simulink model "tesv"  (R2012b)
settings: Solver=ode45  SolverMode=SingleTasking  StartTime=0.0  StopTime=10.0  RelTol=1e-3
libraries: xbsIndex_r4 x837
(part 2 of 6)

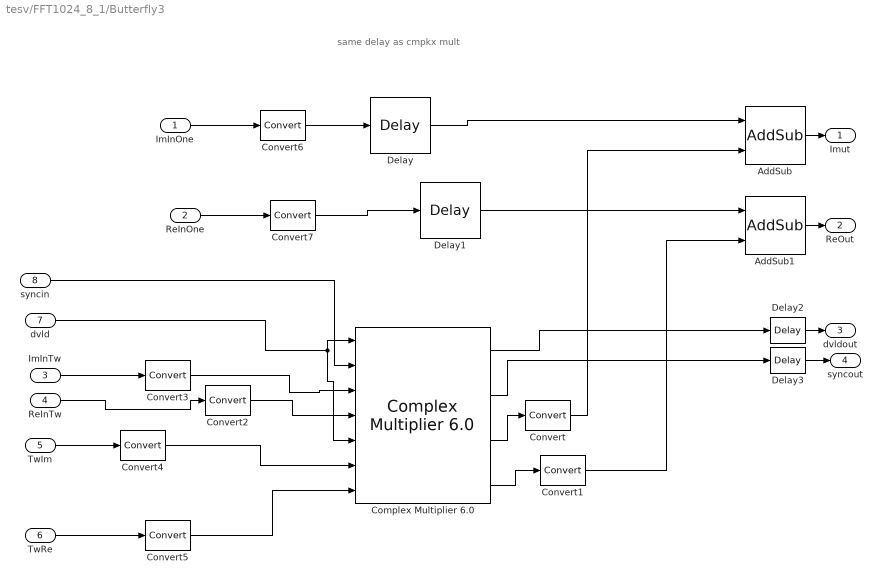
== system tesv/FFT1024_8_1/Butterfly3 ==
  note: same delay as cmpkx mult
  ImInOne : Inport
  ReInOne : Inport  Port=2
  ImInTw : Inport  Port=3
  ReInTw : Inport  Port=4
  TwIm : Inport  Port=5
  TwRe : Inport  Port=6
  dvld : Inport  Port=7
  syncin : Inport  Port=8
  AddSub : xbsIndex_r4/AddSub  mode=Addition  use_carryin=off  use_carryout=off  en=off  latency=1  precision=Full  arith_type=Unsigned  n_bits=16  bin_pt=14  quantization=Truncate  overflow=Wrap  use_behavioral_HDL=off  hw_selection=Fabric  pipelined=off  dbl_ovrd=off  block_type=addsub
  AddSub1 : xbsIndex_r4/AddSub  mode=Addition  use_carryin=off  use_carryout=off  en=off  latency=1  precision=Full  arith_type=Unsigned  n_bits=16  bin_pt=14  quantization=Truncate  overflow=Wrap  use_behavioral_HDL=off  hw_selection=Fabric  pipelined=off  dbl_ovrd=off  block_type=addsub
  "Complex Multiplier 6.0 " : xbsIndex_r4/Complex Multiplier 6.0   hasatlast=on  hasatuser=off  atuserwidth=1  hasbtlast=off  hasbtuser=off  btuserwidth=1  multtype=Use_Mults  optimizegoal=Resources  flowcontrol=NonBlocking  outputwidth=18  roundmode=Truncate  hasctrltlast=off  hasctrltuser=off  ctrltuserwidth=1  outtlastbehv=Pass_A_TLAST  latencyconfig=Automatic  minimumlatency=37  aclken=off  aresetn=off  trim_axipin_name=on  simulation_type=hybrid_sim  simulation_model=sysgen:cmpy_v6_0  data_path_portlist={ 's_axis_a_tdata_real', 's_axis_a_tdata_imag', 's_axis_b_tdata_real', 's_axis_b_tdata_imag', 's_axis_ctrl_tdata_rounding_bit', 'm_axis_dout_tdata_real', 'm_axis_dout_tdata_imag' }  aportwidth=63  bportwidth=63  ip_name=Complex Multiplier  ip_version=6.0  dsptool_ready=true  ipcore_usecache=true  ipcore_useipmodelcache=true  ipcore_verbose=false  ipcore_latency_parameter='minimumlatency'  wrapper_available=true  port_translation_map={ 'aclken' => 'en', 'aresetn' => 'rst'}  block_type=cmpy_v6_0
  Convert{,1..7} (8 alike) : xbsIndex_r4/Convert  gui_display_data_type=Fixed-point  arith_type="Signed  (2's comp)"  n_bits=16  bin_pt=14  float_type=Single  exp_bits=8  fraction_bits=24  quantization=Truncate  overflow=Wrap  en=off  latency=0  pipeline=off  dbl_ovrd=off  block_type=convert
  Delay : xbsIndex_r4/Delay  rst=off  infoeditControl=Selection of Reset will increase slice count due to use of real FFs and instead of SRLs  en=off  latency=6  reg_retiming=off  dbl_ovrd=off  block_type=delay
  Delay1 : xbsIndex_r4/Delay  rst=off  infoeditControl=Selection of Reset will increase slice count due to use of real FFs and instead of SRLs  en=off  latency=6  reg_retiming=off  dbl_ovrd=off  block_type=delay
  Delay2 : xbsIndex_r4/Delay  rst=off  infoeditControl=Selection of Reset will increase slice count due to use of real FFs and instead of SRLs  en=off  latency=1  reg_retiming=off  dbl_ovrd=off  block_type=delay
  Delay3 : xbsIndex_r4/Delay  rst=off  infoeditControl=Selection of Reset will increase slice count due to use of real FFs and instead of SRLs  en=off  latency=1  reg_retiming=off  dbl_ovrd=off  block_type=delay
  Imut : Outport
  ReOut : Outport  Port=2
  dvldout : Outport  Port=3
  syncout : Outport  Port=4
  wires:
  ReInOne/1 -> Convert7/1
  ImInOne/1 -> Convert6/1
  AddSub/1 -> Imut/1
  AddSub1/1 -> ReOut/1
  ImInTw/1 -> Convert3/1
  ReInTw/1 -> Convert2/1
  Delay/1 -> AddSub/1
  Delay1/1 -> AddSub1/1
  TwIm/1 -> Convert4/1
  TwRe/1 -> Convert5/1
  dvld/1 -> "Complex Multiplier 6.0 "/1, "Complex Multiplier 6.0 "/5
  Convert6/1 -> Delay/1
  Convert7/1 -> Delay1/1
  Convert3/1 -> "Complex Multiplier 6.0 "/3
  Convert2/1 -> "Complex Multiplier 6.0 "/4
  Convert4/1 -> "Complex Multiplier 6.0 "/6
  Convert5/1 -> "Complex Multiplier 6.0 "/7
  Convert1/1 -> AddSub1/2
  syncin/1 -> "Complex Multiplier 6.0 "/2
  "Complex Multiplier 6.0 "/4 -> Convert1/1
  "Complex Multiplier 6.0 "/3 -> Convert/1
  "Complex Multiplier 6.0 "/1 -> Delay2/1
  "Complex Multiplier 6.0 "/2 -> Delay3/1
  Convert/1 -> AddSub/2
  Delay2/1 -> dvldout/1
  Delay3/1 -> syncout/1

== system tesv/FFT1024_8_1/Butterfly4 ==
  note: same delay as cmpkx mult
  ImInOne : Inport
  ReInOne : Inport  Port=2
  ImInTw : Inport  Port=3
  ReInTw : Inport  Port=4
  TwIm : Inport  Port=5
  TwRe : Inport  Port=6
  dvld : Inport  Port=7
  syncin : Inport  Port=8
  AddSub : xbsIndex_r4/AddSub  mode=Addition  use_carryin=off  use_carryout=off  en=off  latency=1  precision=Full  arith_type=Unsigned  n_bits=16  bin_pt=14  quantization=Truncate  overflow=Wrap  use_behavioral_HDL=off  hw_selection=Fabric  pipelined=off  dbl_ovrd=off  block_type=addsub
  AddSub1 : xbsIndex_r4/AddSub  mode=Addition  use_carryin=off  use_carryout=off  en=off  latency=1  precision=Full  arith_type=Unsigned  n_bits=16  bin_pt=14  quantization=Truncate  overflow=Wrap  use_behavioral_HDL=off  hw_selection=Fabric  pipelined=off  dbl_ovrd=off  block_type=addsub
  "Complex Multiplier 6.0 " : xbsIndex_r4/Complex Multiplier 6.0   hasatlast=on  hasatuser=off  atuserwidth=1  hasbtlast=off  hasbtuser=off  btuserwidth=1  multtype=Use_Mults  optimizegoal=Resources  flowcontrol=NonBlocking  outputwidth=18  roundmode=Truncate  hasctrltlast=off  hasctrltuser=off  ctrltuserwidth=1  outtlastbehv=Pass_A_TLAST  latencyconfig=Automatic  minimumlatency=37  aclken=off  aresetn=off  trim_axipin_name=on  simulation_type=hybrid_sim  simulation_model=sysgen:cmpy_v6_0  data_path_portlist={ 's_axis_a_tdata_real', 's_axis_a_tdata_imag', 's_axis_b_tdata_real', 's_axis_b_tdata_imag', 's_axis_ctrl_tdata_rounding_bit', 'm_axis_dout_tdata_real', 'm_axis_dout_tdata_imag' }  aportwidth=63  bportwidth=63  ip_name=Complex Multiplier  ip_version=6.0  dsptool_ready=true  ipcore_usecache=true  ipcore_useipmodelcache=true  ipcore_verbose=false  ipcore_latency_parameter='minimumlatency'  wrapper_available=true  port_translation_map={ 'aclken' => 'en', 'aresetn' => 'rst'}  block_type=cmpy_v6_0
  Convert{,1..7} (8 alike) : xbsIndex_r4/Convert  gui_display_data_type=Fixed-point  arith_type="Signed  (2's comp)"  n_bits=16  bin_pt=14  float_type=Single  exp_bits=8  fraction_bits=24  quantization=Truncate  overflow=Wrap  en=off  latency=0  pipeline=off  dbl_ovrd=off  block_type=convert
  Delay : xbsIndex_r4/Delay  rst=off  infoeditControl=Selection of Reset will increase slice count due to use of real FFs and instead of SRLs  en=off  latency=6  reg_retiming=off  dbl_ovrd=off  block_type=delay
  Delay1 : xbsIndex_r4/Delay  rst=off  infoeditControl=Selection of Reset will increase slice count due to use of real FFs and instead of SRLs  en=off  latency=6  reg_retiming=off  dbl_ovrd=off  block_type=delay
  Delay2 : xbsIndex_r4/Delay  rst=off  infoeditControl=Selection of Reset will increase slice count due to use of real FFs and instead of SRLs  en=off  latency=1  reg_retiming=off  dbl_ovrd=off  block_type=delay
  Delay3 : xbsIndex_r4/Delay  rst=off  infoeditControl=Selection of Reset will increase slice count due to use of real FFs and instead of SRLs  en=off  latency=1  reg_retiming=off  dbl_ovrd=off  block_type=delay
  Imut : Outport
  ReOut : Outport  Port=2
  dvldout : Outport  Port=3
  syncout : Outport  Port=4
  wires:
  ReInOne/1 -> Convert7/1
  ImInOne/1 -> Convert6/1
  AddSub/1 -> Imut/1
  AddSub1/1 -> ReOut/1
  ImInTw/1 -> Convert3/1
  ReInTw/1 -> Convert2/1
  Delay/1 -> AddSub/1
  Delay1/1 -> AddSub1/1
  TwIm/1 -> Convert4/1
  TwRe/1 -> Convert5/1
  dvld/1 -> "Complex Multiplier 6.0 "/1, "Complex Multiplier 6.0 "/5
  Convert6/1 -> Delay/1
  Convert7/1 -> Delay1/1
  Convert3/1 -> "Complex Multiplier 6.0 "/3
  Convert2/1 -> "Complex Multiplier 6.0 "/4
  Convert4/1 -> "Complex Multiplier 6.0 "/6
  Convert5/1 -> "Complex Multiplier 6.0 "/7
  Convert1/1 -> AddSub1/2
  syncin/1 -> "Complex Multiplier 6.0 "/2
  "Complex Multiplier 6.0 "/4 -> Convert1/1
  "Complex Multiplier 6.0 "/3 -> Convert/1
  "Complex Multiplier 6.0 "/1 -> Delay2/1
  "Complex Multiplier 6.0 "/2 -> Delay3/1
  Convert/1 -> AddSub/2
  Delay2/1 -> dvldout/1
  Delay3/1 -> syncout/1

== system tesv/FFT1024_8_1/Butterfly5 ==
  note: same delay as cmpkx mult
  ImInOne : Inport
  ReInOne : Inport  Port=2
  ImInTw : Inport  Port=3
  ReInTw : Inport  Port=4
  TwIm : Inport  Port=5
  TwRe : Inport  Port=6
  dvld : Inport  Port=7
  syncin : Inport  Port=8
  AddSub : xbsIndex_r4/AddSub  mode=Addition  use_carryin=off  use_carryout=off  en=off  latency=1  precision=Full  arith_type=Unsigned  n_bits=16  bin_pt=14  quantization=Truncate  overflow=Wrap  use_behavioral_HDL=off  hw_selection=Fabric  pipelined=off  dbl_ovrd=off  block_type=addsub
  AddSub1 : xbsIndex_r4/AddSub  mode=Addition  use_carryin=off  use_carryout=off  en=off  latency=1  precision=Full  arith_type=Unsigned  n_bits=16  bin_pt=14  quantization=Truncate  overflow=Wrap  use_behavioral_HDL=off  hw_selection=Fabric  pipelined=off  dbl_ovrd=off  block_type=addsub
  "Complex Multiplier 6.0 " : xbsIndex_r4/Complex Multiplier 6.0   hasatlast=on  hasatuser=off  atuserwidth=1  hasbtlast=off  hasbtuser=off  btuserwidth=1  multtype=Use_Mults  optimizegoal=Resources  flowcontrol=NonBlocking  outputwidth=18  roundmode=Truncate  hasctrltlast=off  hasctrltuser=off  ctrltuserwidth=1  outtlastbehv=Pass_A_TLAST  latencyconfig=Automatic  minimumlatency=37  aclken=off  aresetn=off  trim_axipin_name=on  simulation_type=hybrid_sim  simulation_model=sysgen:cmpy_v6_0  data_path_portlist={ 's_axis_a_tdata_real', 's_axis_a_tdata_imag', 's_axis_b_tdata_real', 's_axis_b_tdata_imag', 's_axis_ctrl_tdata_rounding_bit', 'm_axis_dout_tdata_real', 'm_axis_dout_tdata_imag' }  aportwidth=63  bportwidth=63  ip_name=Complex Multiplier  ip_version=6.0  dsptool_ready=true  ipcore_usecache=true  ipcore_useipmodelcache=true  ipcore_verbose=false  ipcore_latency_parameter='minimumlatency'  wrapper_available=true  port_translation_map={ 'aclken' => 'en', 'aresetn' => 'rst'}  block_type=cmpy_v6_0
  Convert{,1..7} (8 alike) : xbsIndex_r4/Convert  gui_display_data_type=Fixed-point  arith_type="Signed  (2's comp)"  n_bits=16  bin_pt=14  float_type=Single  exp_bits=8  fraction_bits=24  quantization=Truncate  overflow=Wrap  en=off  latency=0  pipeline=off  dbl_ovrd=off  block_type=convert
  Delay : xbsIndex_r4/Delay  rst=off  infoeditControl=Selection of Reset will increase slice count due to use of real FFs and instead of SRLs  en=off  latency=6  reg_retiming=off  dbl_ovrd=off  block_type=delay
  Delay1 : xbsIndex_r4/Delay  rst=off  infoeditControl=Selection of Reset will increase slice count due to use of real FFs and instead of SRLs  en=off  latency=6  reg_retiming=off  dbl_ovrd=off  block_type=delay
  Delay2 : xbsIndex_r4/Delay  rst=off  infoeditControl=Selection of Reset will increase slice count due to use of real FFs and instead of SRLs  en=off  latency=1  reg_retiming=off  dbl_ovrd=off  block_type=delay
  Delay3 : xbsIndex_r4/Delay  rst=off  infoeditControl=Selection of Reset will increase slice count due to use of real FFs and instead of SRLs  en=off  latency=1  reg_retiming=off  dbl_ovrd=off  block_type=delay
  Imut : Outport
  ReOut : Outport  Port=2
  dvldout : Outport  Port=3
  syncout : Outport  Port=4
  wires:
  ReInOne/1 -> Convert7/1
  ImInOne/1 -> Convert6/1
  AddSub/1 -> Imut/1
  AddSub1/1 -> ReOut/1
  ImInTw/1 -> Convert3/1
  ReInTw/1 -> Convert2/1
  Delay/1 -> AddSub/1
  Delay1/1 -> AddSub1/1
  TwIm/1 -> Convert4/1
  TwRe/1 -> Convert5/1
  dvld/1 -> "Complex Multiplier 6.0 "/1, "Complex Multiplier 6.0 "/5
  Convert6/1 -> Delay/1
  Convert7/1 -> Delay1/1
  Convert3/1 -> "Complex Multiplier 6.0 "/3
  Convert2/1 -> "Complex Multiplier 6.0 "/4
  Convert4/1 -> "Complex Multiplier 6.0 "/6
  Convert5/1 -> "Complex Multiplier 6.0 "/7
  Convert1/1 -> AddSub1/2
  syncin/1 -> "Complex Multiplier 6.0 "/2
  "Complex Multiplier 6.0 "/4 -> Convert1/1
  "Complex Multiplier 6.0 "/3 -> Convert/1
  "Complex Multiplier 6.0 "/1 -> Delay2/1
  "Complex Multiplier 6.0 "/2 -> Delay3/1
  Convert/1 -> AddSub/2
  Delay2/1 -> dvldout/1
  Delay3/1 -> syncout/1

== system tesv/FFT1024_8_1/Butterfly6 ==
  note: same delay as cmpkx mult
  ImInOne : Inport
  ReInOne : Inport  Port=2
  ImInTw : Inport  Port=3
  ReInTw : Inport  Port=4
  TwIm : Inport  Port=5
  TwRe : Inport  Port=6
  dvld : Inport  Port=7
  syncin : Inport  Port=8
  AddSub : xbsIndex_r4/AddSub  mode=Addition  use_carryin=off  use_carryout=off  en=off  latency=1  precision=Full  arith_type=Unsigned  n_bits=16  bin_pt=14  quantization=Truncate  overflow=Wrap  use_behavioral_HDL=off  hw_selection=Fabric  pipelined=off  dbl_ovrd=off  block_type=addsub
  AddSub1 : xbsIndex_r4/AddSub  mode=Addition  use_carryin=off  use_carryout=off  en=off  latency=1  precision=Full  arith_type=Unsigned  n_bits=16  bin_pt=14  quantization=Truncate  overflow=Wrap  use_behavioral_HDL=off  hw_selection=Fabric  pipelined=off  dbl_ovrd=off  block_type=addsub
  "Complex Multiplier 6.0 " : xbsIndex_r4/Complex Multiplier 6.0   hasatlast=on  hasatuser=off  atuserwidth=1  hasbtlast=off  hasbtuser=off  btuserwidth=1  multtype=Use_Mults  optimizegoal=Resources  flowcontrol=NonBlocking  outputwidth=18  roundmode=Truncate  hasctrltlast=off  hasctrltuser=off  ctrltuserwidth=1  outtlastbehv=Pass_A_TLAST  latencyconfig=Automatic  minimumlatency=37  aclken=off  aresetn=off  trim_axipin_name=on  simulation_type=hybrid_sim  simulation_model=sysgen:cmpy_v6_0  data_path_portlist={ 's_axis_a_tdata_real', 's_axis_a_tdata_imag', 's_axis_b_tdata_real', 's_axis_b_tdata_imag', 's_axis_ctrl_tdata_rounding_bit', 'm_axis_dout_tdata_real', 'm_axis_dout_tdata_imag' }  aportwidth=63  bportwidth=63  ip_name=Complex Multiplier  ip_version=6.0  dsptool_ready=true  ipcore_usecache=true  ipcore_useipmodelcache=true  ipcore_verbose=false  ipcore_latency_parameter='minimumlatency'  wrapper_available=true  port_translation_map={ 'aclken' => 'en', 'aresetn' => 'rst'}  block_type=cmpy_v6_0
  Convert{,1..7} (8 alike) : xbsIndex_r4/Convert  gui_display_data_type=Fixed-point  arith_type="Signed  (2's comp)"  n_bits=16  bin_pt=14  float_type=Single  exp_bits=8  fraction_bits=24  quantization=Truncate  overflow=Wrap  en=off  latency=0  pipeline=off  dbl_ovrd=off  block_type=convert
  Delay : xbsIndex_r4/Delay  rst=off  infoeditControl=Selection of Reset will increase slice count due to use of real FFs and instead of SRLs  en=off  latency=6  reg_retiming=off  dbl_ovrd=off  block_type=delay
  Delay1 : xbsIndex_r4/Delay  rst=off  infoeditControl=Selection of Reset will increase slice count due to use of real FFs and instead of SRLs  en=off  latency=6  reg_retiming=off  dbl_ovrd=off  block_type=delay
  Delay2 : xbsIndex_r4/Delay  rst=off  infoeditControl=Selection of Reset will increase slice count due to use of real FFs and instead of SRLs  en=off  latency=1  reg_retiming=off  dbl_ovrd=off  block_type=delay
  Delay3 : xbsIndex_r4/Delay  rst=off  infoeditControl=Selection of Reset will increase slice count due to use of real FFs and instead of SRLs  en=off  latency=1  reg_retiming=off  dbl_ovrd=off  block_type=delay
  Imut : Outport
  ReOut : Outport  Port=2
  dvldout : Outport  Port=3
  syncout : Outport  Port=4
  wires:
  ReInOne/1 -> Convert7/1
  ImInOne/1 -> Convert6/1
  AddSub/1 -> Imut/1
  AddSub1/1 -> ReOut/1
  ImInTw/1 -> Convert3/1
  ReInTw/1 -> Convert2/1
  Delay/1 -> AddSub/1
  Delay1/1 -> AddSub1/1
  TwIm/1 -> Convert4/1
  TwRe/1 -> Convert5/1
  dvld/1 -> "Complex Multiplier 6.0 "/1, "Complex Multiplier 6.0 "/5
  Convert6/1 -> Delay/1
  Convert7/1 -> Delay1/1
  Convert3/1 -> "Complex Multiplier 6.0 "/3
  Convert2/1 -> "Complex Multiplier 6.0 "/4
  Convert4/1 -> "Complex Multiplier 6.0 "/6
  Convert5/1 -> "Complex Multiplier 6.0 "/7
  Convert1/1 -> AddSub1/2
  syncin/1 -> "Complex Multiplier 6.0 "/2
  "Complex Multiplier 6.0 "/4 -> Convert1/1
  "Complex Multiplier 6.0 "/3 -> Convert/1
  "Complex Multiplier 6.0 "/1 -> Delay2/1
  "Complex Multiplier 6.0 "/2 -> Delay3/1
  Convert/1 -> AddSub/2
  Delay2/1 -> dvldout/1
  Delay3/1 -> syncout/1

== system tesv/FFT1024_8_1/Butterfly7 ==
  note: same delay as cmpkx mult
  ImInOne : Inport
  ReInOne : Inport  Port=2
  ImInTw : Inport  Port=3
  ReInTw : Inport  Port=4
  TwIm : Inport  Port=5
  TwRe : Inport  Port=6
  dvld : Inport  Port=7
  syncin : Inport  Port=8
  AddSub : xbsIndex_r4/AddSub  mode=Addition  use_carryin=off  use_carryout=off  en=off  latency=1  precision=Full  arith_type=Unsigned  n_bits=16  bin_pt=14  quantization=Truncate  overflow=Wrap  use_behavioral_HDL=off  hw_selection=Fabric  pipelined=off  dbl_ovrd=off  block_type=addsub
  AddSub1 : xbsIndex_r4/AddSub  mode=Addition  use_carryin=off  use_carryout=off  en=off  latency=1  precision=Full  arith_type=Unsigned  n_bits=16  bin_pt=14  quantization=Truncate  overflow=Wrap  use_behavioral_HDL=off  hw_selection=Fabric  pipelined=off  dbl_ovrd=off  block_type=addsub
  "Complex Multiplier 6.0 " : xbsIndex_r4/Complex Multiplier 6.0   hasatlast=on  hasatuser=off  atuserwidth=1  hasbtlast=off  hasbtuser=off  btuserwidth=1  multtype=Use_Mults  optimizegoal=Resources  flowcontrol=NonBlocking  outputwidth=18  roundmode=Truncate  hasctrltlast=off  hasctrltuser=off  ctrltuserwidth=1  outtlastbehv=Pass_A_TLAST  latencyconfig=Automatic  minimumlatency=37  aclken=off  aresetn=off  trim_axipin_name=on  simulation_type=hybrid_sim  simulation_model=sysgen:cmpy_v6_0  data_path_portlist={ 's_axis_a_tdata_real', 's_axis_a_tdata_imag', 's_axis_b_tdata_real', 's_axis_b_tdata_imag', 's_axis_ctrl_tdata_rounding_bit', 'm_axis_dout_tdata_real', 'm_axis_dout_tdata_imag' }  aportwidth=63  bportwidth=63  ip_name=Complex Multiplier  ip_version=6.0  dsptool_ready=true  ipcore_usecache=true  ipcore_useipmodelcache=true  ipcore_verbose=false  ipcore_latency_parameter='minimumlatency'  wrapper_available=true  port_translation_map={ 'aclken' => 'en', 'aresetn' => 'rst'}  block_type=cmpy_v6_0
  Convert{,1..7} (8 alike) : xbsIndex_r4/Convert  gui_display_data_type=Fixed-point  arith_type="Signed  (2's comp)"  n_bits=16  bin_pt=14  float_type=Single  exp_bits=8  fraction_bits=24  quantization=Truncate  overflow=Wrap  en=off  latency=0  pipeline=off  dbl_ovrd=off  block_type=convert
  Delay : xbsIndex_r4/Delay  rst=off  infoeditControl=Selection of Reset will increase slice count due to use of real FFs and instead of SRLs  en=off  latency=6  reg_retiming=off  dbl_ovrd=off  block_type=delay
  Delay1 : xbsIndex_r4/Delay  rst=off  infoeditControl=Selection of Reset will increase slice count due to use of real FFs and instead of SRLs  en=off  latency=6  reg_retiming=off  dbl_ovrd=off  block_type=delay
  Delay2 : xbsIndex_r4/Delay  rst=off  infoeditControl=Selection of Reset will increase slice count due to use of real FFs and instead of SRLs  en=off  latency=1  reg_retiming=off  dbl_ovrd=off  block_type=delay
  Delay3 : xbsIndex_r4/Delay  rst=off  infoeditControl=Selection of Reset will increase slice count due to use of real FFs and instead of SRLs  en=off  latency=1  reg_retiming=off  dbl_ovrd=off  block_type=delay
  Imut : Outport
  ReOut : Outport  Port=2
  dvldout : Outport  Port=3
  syncout : Outport  Port=4
  wires:
  ReInOne/1 -> Convert7/1
  ImInOne/1 -> Convert6/1
  AddSub/1 -> Imut/1
  AddSub1/1 -> ReOut/1
  ImInTw/1 -> Convert3/1
  ReInTw/1 -> Convert2/1
  Delay/1 -> AddSub/1
  Delay1/1 -> AddSub1/1
  TwIm/1 -> Convert4/1
  TwRe/1 -> Convert5/1
  dvld/1 -> "Complex Multiplier 6.0 "/1, "Complex Multiplier 6.0 "/5
  Convert6/1 -> Delay/1
  Convert7/1 -> Delay1/1
  Convert3/1 -> "Complex Multiplier 6.0 "/3
  Convert2/1 -> "Complex Multiplier 6.0 "/4
  Convert4/1 -> "Complex Multiplier 6.0 "/6
  Convert5/1 -> "Complex Multiplier 6.0 "/7
  Convert1/1 -> AddSub1/2
  syncin/1 -> "Complex Multiplier 6.0 "/2
  "Complex Multiplier 6.0 "/4 -> Convert1/1
  "Complex Multiplier 6.0 "/3 -> Convert/1
  "Complex Multiplier 6.0 "/1 -> Delay2/1
  "Complex Multiplier 6.0 "/2 -> Delay3/1
  Convert/1 -> AddSub/2
  Delay2/1 -> dvldout/1
  Delay3/1 -> syncout/1

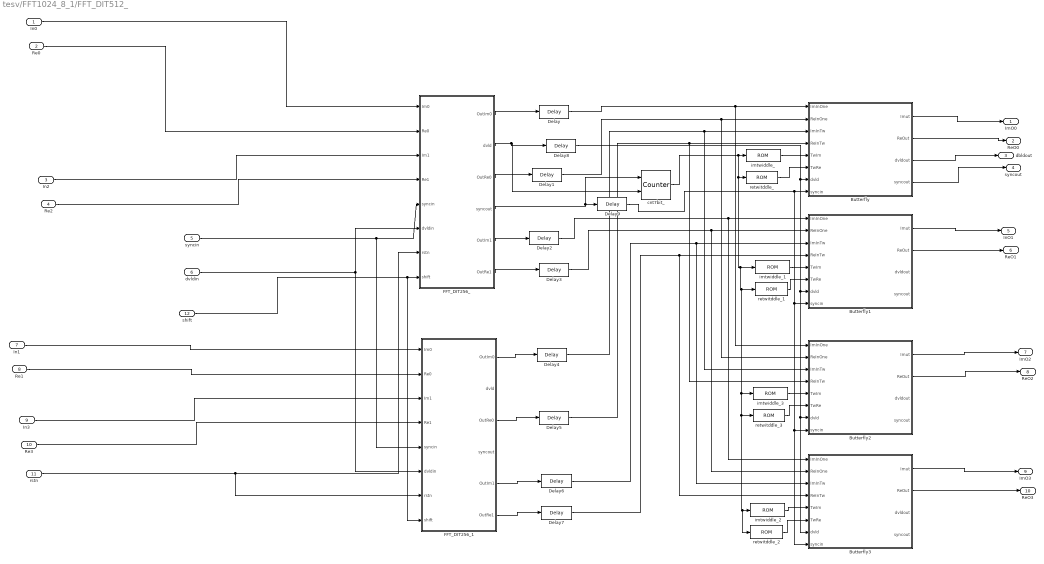
== system tesv/FFT1024_8_1/FFT_DIT512_ ==
  In0 : Inport
  Re0 : Inport  Port=2
  In2 : Inport  Port=3
  Re2 : Inport  Port=4
  syncin : Inport  Port=5
  dvldin : Inport  Port=6
  In1 : Inport  Port=7
  Re1 : Inport  Port=8
  In3 : Inport  Port=9
  Re3 : Inport  Port=10
  rstn : Inport  Port=11
  shift : Inport  Port=12
  Butterfly : Subsystem
  Butterfly1 : Subsystem
  Butterfly2 : Subsystem
  Butterfly3 : Subsystem
  Delay{,1..9} (10 alike) : xbsIndex_r4/Delay  rst=off  infoeditControl=Selection of Reset will increase slice count due to use of real FFs and instead of SRLs  en=off  latency=1  reg_retiming=off  dbl_ovrd=off  block_type=delay
  FFT_DIT256_ : Subsystem
  FFT_DIT256_1 : Subsystem
  cnt7bit_ : xbsIndex_r4/Counter  cnt_type=Free Running  cnt_to=Inf  operation=Up  start_count=0  cnt_by_val=1  arith_type=Unsigned  n_bits=7  bin_pt=0  load_pin=off  rst=on  en=on  explicit_period=on  period=1  use_behavioral_HDL=off  implementation=Fabric  dbl_ovrd=off  block_type=counter
  imtwiddle_ : xbsIndex_r4/ROM  depth=128  initVector=-sin(2*pi*(0:127)/512)  distributed_mem=Block RAM  rst=off  init_reg=0  en=off  latency=1  gui_display_data_type=Fixed-point  arith_type="Signed  (2's comp)"  n_bits=16  bin_pt=15  preci_type=Single  exp_width=8  frac_width=24  optimize=Area  use_rpm=on  dbl_ovrd=off  block_type=sprom
  imtwiddle_1 : xbsIndex_r4/ROM  depth=128  initVector=-sin(2*pi*(128:255)/512)  distributed_mem=Block RAM  rst=off  init_reg=0  en=off  latency=1  gui_display_data_type=Fixed-point  arith_type="Signed  (2's comp)"  n_bits=16  bin_pt=15  preci_type=Single  exp_width=8  frac_width=24  optimize=Area  use_rpm=on  dbl_ovrd=off  block_type=sprom
  imtwiddle_2 : xbsIndex_r4/ROM  depth=128  initVector=-sin(2*pi*(384:511)/512)  distributed_mem=Block RAM  rst=off  init_reg=0  en=off  latency=1  gui_display_data_type=Fixed-point  arith_type="Signed  (2's comp)"  n_bits=16  bin_pt=15  preci_type=Single  exp_width=8  frac_width=24  optimize=Area  use_rpm=on  dbl_ovrd=off  block_type=sprom
  imtwiddle_3 : xbsIndex_r4/ROM  depth=128  initVector=-sin(2*pi*(256:383)/512)  distributed_mem=Block RAM  rst=off  init_reg=0  en=off  latency=1  gui_display_data_type=Fixed-point  arith_type="Signed  (2's comp)"  n_bits=16  bin_pt=15  preci_type=Single  exp_width=8  frac_width=24  optimize=Area  use_rpm=on  dbl_ovrd=off  block_type=sprom
  retwitddle_ : xbsIndex_r4/ROM  depth=128  initVector=cos(2*pi*(0:127)/512)  distributed_mem=Block RAM  rst=off  init_reg=0  en=off  latency=1  gui_display_data_type=Fixed-point  arith_type="Signed  (2's comp)"  n_bits=16  bin_pt=14  preci_type=Single  exp_width=8  frac_width=24  optimize=Area  use_rpm=on  dbl_ovrd=off  block_type=sprom
  retwitddle_1 : xbsIndex_r4/ROM  depth=128  initVector=cos(2*pi*(128:255)/512)  distributed_mem=Block RAM  rst=off  init_reg=0  en=off  latency=1  gui_display_data_type=Fixed-point  arith_type="Signed  (2's comp)"  n_bits=16  bin_pt=14  preci_type=Single  exp_width=8  frac_width=24  optimize=Area  use_rpm=on  dbl_ovrd=off  block_type=sprom
  retwitddle_2 : xbsIndex_r4/ROM  depth=128  initVector=cos(2*pi*(384:511)/512)  distributed_mem=Block RAM  rst=off  init_reg=0  en=off  latency=1  gui_display_data_type=Fixed-point  arith_type="Signed  (2's comp)"  n_bits=16  bin_pt=14  preci_type=Single  exp_width=8  frac_width=24  optimize=Area  use_rpm=on  dbl_ovrd=off  block_type=sprom
  retwitddle_3 : xbsIndex_r4/ROM  depth=128  initVector=cos(2*pi*(256:383)/512)  distributed_mem=Block RAM  rst=off  init_reg=0  en=off  latency=1  gui_display_data_type=Fixed-point  arith_type="Signed  (2's comp)"  n_bits=16  bin_pt=14  preci_type=Single  exp_width=8  frac_width=24  optimize=Area  use_rpm=on  dbl_ovrd=off  block_type=sprom
  ImO0 : Outport
  ReO0 : Outport  Port=2
  dbldout : Outport  Port=3
  syncout : Outport  Port=4
  InO1 : Outport  Port=5
  ReO1 : Outport  Port=6
  ImO2 : Outport  Port=7
  ReO2 : Outport  Port=8
  ImO3 : Outport  Port=9
  ReO3 : Outport  Port=10
  wires:
  Delay1/1 -> Butterfly2/2(ReInOne), Butterfly/2(ReInOne)
  FFT_DIT256_1/1(OutIm0) -> Delay4/1
  In1/1 -> FFT_DIT256_1/1(Im0)
  Butterfly1/2(ReOut) -> ReO1/1
  FFT_DIT256_/3(OutRe0) -> Delay1/1
  FFT_DIT256_/2(dvld) -> Delay8/1, cnt7bit_/2
  Butterfly2/1(Imut) -> ImO2/1
  Delay3/1 -> Butterfly3/2(ReInOne), Butterfly1/2(ReInOne)
  In3/1 -> FFT_DIT256_1/3(Im1)
  retwitddle_1/1 -> Butterfly1/6(TwRe)
  dvldin/1 -> FFT_DIT256_1/6(dvldin), FFT_DIT256_/6(dvldin)
  FFT_DIT256_1/3(OutRe0) -> Delay5/1
  Re3/1 -> FFT_DIT256_1/4(Re1)
  Delay5/1 -> Butterfly2/4(ReInTw), Butterfly/4(ReInTw)
  cnt7bit_/1 -> retwitddle_2/1, imtwiddle_2/1, retwitddle_3/1, imtwiddle_3/1, retwitddle_1/1, imtwiddle_1/1, retwitddle_/1, imtwiddle_/1
  Delay6/1 -> Butterfly3/3(ImInTw), Butterfly1/3(ImInTw)
  imtwiddle_2/1 -> Butterfly3/5(TwIm)
  Delay4/1 -> Butterfly2/3(ImInTw), Butterfly/3(ImInTw)
  retwitddle_2/1 -> Butterfly3/6(TwRe)
  Re2/1 -> FFT_DIT256_/4(Re1)
  Re0/1 -> FFT_DIT256_/2(Re0)
  Butterfly/3(dvldout) -> dbldout/1
  Delay/1 -> Butterfly2/1(ImInOne), Butterfly/1(ImInOne)
  Butterfly3/1(Imut) -> ImO3/1
  retwitddle_3/1 -> Butterfly2/6(TwRe)
  imtwiddle_/1 -> Butterfly/5(TwIm)
  imtwiddle_3/1 -> Butterfly2/5(TwIm)
  FFT_DIT256_/1(OutIm0) -> Delay/1
  Butterfly3/2(ReOut) -> ReO3/1
  Butterfly/1(Imut) -> ImO0/1
  Butterfly/2(ReOut) -> ReO0/1
  FFT_DIT256_1/6(OutRe1) -> Delay7/1
  Delay9/1 -> Butterfly/8(syncin), Butterfly1/8(syncin), Butterfly3/8(syncin), Butterfly2/8(syncin)
  FFT_DIT256_1/5(OutIm1) -> Delay6/1
  Butterfly1/1(Imut) -> InO1/1
  imtwiddle_1/1 -> Butterfly1/5(TwIm)
  Re1/1 -> FFT_DIT256_1/2(Re0)
  Butterfly/4(syncout) -> syncout/1
  FFT_DIT256_/6(OutRe1) -> Delay3/1
  In0/1 -> FFT_DIT256_/1(Im0)
  Delay7/1 -> Butterfly3/4(ReInTw), Butterfly1/4(ReInTw)
  Butterfly2/2(ReOut) -> ReO2/1
  FFT_DIT256_/4(syncout) -> Delay9/1, cnt7bit_/1
  Delay8/1 -> Butterfly/7(dvld), Butterfly1/7(dvld), Butterfly3/7(dvld), Butterfly2/7(dvld)
  FFT_DIT256_/5(OutIm1) -> Delay2/1
  retwitddle_/1 -> Butterfly/6(TwRe)
  In2/1 -> FFT_DIT256_/3(Im1)
  syncin/1 -> FFT_DIT256_1/5(syncin), FFT_DIT256_/5(syncin)
  Delay2/1 -> Butterfly3/1(ImInOne), Butterfly1/1(ImInOne)
  rstn/1 -> FFT_DIT256_1/7(rstn), FFT_DIT256_/7(rstn)
  shift/1 -> FFT_DIT256_1/8(shift), FFT_DIT256_/8(shift)

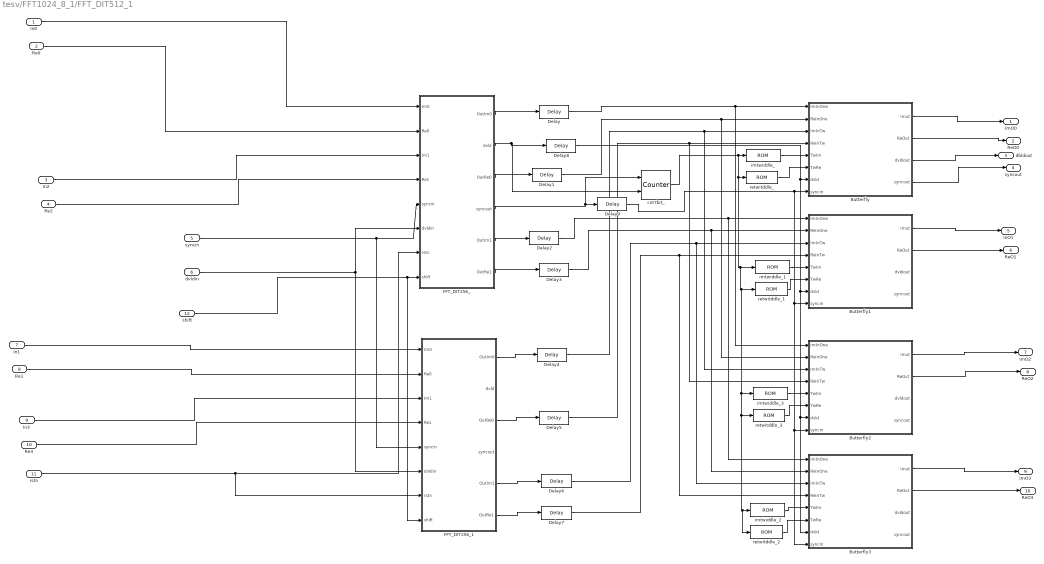
== system tesv/FFT1024_8_1/FFT_DIT512_1 ==
  In0 : Inport
  Re0 : Inport  Port=2
  In2 : Inport  Port=3
  Re2 : Inport  Port=4
  syncin : Inport  Port=5
  dvldin : Inport  Port=6
  In1 : Inport  Port=7
  Re1 : Inport  Port=8
  In3 : Inport  Port=9
  Re3 : Inport  Port=10
  rstn : Inport  Port=11
  shift : Inport  Port=12
  Butterfly : Subsystem
  Butterfly1 : Subsystem
  Butterfly2 : Subsystem
  Butterfly3 : Subsystem
  Delay{,1..9} (10 alike) : xbsIndex_r4/Delay  rst=off  infoeditControl=Selection of Reset will increase slice count due to use of real FFs and instead of SRLs  en=off  latency=1  reg_retiming=off  dbl_ovrd=off  block_type=delay
  FFT_DIT256_ : Subsystem
  FFT_DIT256_1 : Subsystem
  cnt7bit_ : xbsIndex_r4/Counter  cnt_type=Free Running  cnt_to=Inf  operation=Up  start_count=0  cnt_by_val=1  arith_type=Unsigned  n_bits=7  bin_pt=0  load_pin=off  rst=on  en=on  explicit_period=on  period=1  use_behavioral_HDL=off  implementation=Fabric  dbl_ovrd=off  block_type=counter
  imtwiddle_ : xbsIndex_r4/ROM  depth=128  initVector=-sin(2*pi*(0:127)/512)  distributed_mem=Block RAM  rst=off  init_reg=0  en=off  latency=1  gui_display_data_type=Fixed-point  arith_type="Signed  (2's comp)"  n_bits=16  bin_pt=15  preci_type=Single  exp_width=8  frac_width=24  optimize=Area  use_rpm=on  dbl_ovrd=off  block_type=sprom
  imtwiddle_1 : xbsIndex_r4/ROM  depth=128  initVector=-sin(2*pi*(128:255)/512)  distributed_mem=Block RAM  rst=off  init_reg=0  en=off  latency=1  gui_display_data_type=Fixed-point  arith_type="Signed  (2's comp)"  n_bits=16  bin_pt=15  preci_type=Single  exp_width=8  frac_width=24  optimize=Area  use_rpm=on  dbl_ovrd=off  block_type=sprom
  imtwiddle_2 : xbsIndex_r4/ROM  depth=128  initVector=-sin(2*pi*(384:511)/512)  distributed_mem=Block RAM  rst=off  init_reg=0  en=off  latency=1  gui_display_data_type=Fixed-point  arith_type="Signed  (2's comp)"  n_bits=16  bin_pt=15  preci_type=Single  exp_width=8  frac_width=24  optimize=Area  use_rpm=on  dbl_ovrd=off  block_type=sprom
  imtwiddle_3 : xbsIndex_r4/ROM  depth=128  initVector=-sin(2*pi*(256:383)/512)  distributed_mem=Block RAM  rst=off  init_reg=0  en=off  latency=1  gui_display_data_type=Fixed-point  arith_type="Signed  (2's comp)"  n_bits=16  bin_pt=15  preci_type=Single  exp_width=8  frac_width=24  optimize=Area  use_rpm=on  dbl_ovrd=off  block_type=sprom
  retwitddle_ : xbsIndex_r4/ROM  depth=128  initVector=cos(2*pi*(0:127)/512)  distributed_mem=Block RAM  rst=off  init_reg=0  en=off  latency=1  gui_display_data_type=Fixed-point  arith_type="Signed  (2's comp)"  n_bits=16  bin_pt=14  preci_type=Single  exp_width=8  frac_width=24  optimize=Area  use_rpm=on  dbl_ovrd=off  block_type=sprom
  retwitddle_1 : xbsIndex_r4/ROM  depth=128  initVector=cos(2*pi*(128:255)/512)  distributed_mem=Block RAM  rst=off  init_reg=0  en=off  latency=1  gui_display_data_type=Fixed-point  arith_type="Signed  (2's comp)"  n_bits=16  bin_pt=14  preci_type=Single  exp_width=8  frac_width=24  optimize=Area  use_rpm=on  dbl_ovrd=off  block_type=sprom
  retwitddle_2 : xbsIndex_r4/ROM  depth=128  initVector=cos(2*pi*(384:511)/512)  distributed_mem=Block RAM  rst=off  init_reg=0  en=off  latency=1  gui_display_data_type=Fixed-point  arith_type="Signed  (2's comp)"  n_bits=16  bin_pt=14  preci_type=Single  exp_width=8  frac_width=24  optimize=Area  use_rpm=on  dbl_ovrd=off  block_type=sprom
  retwitddle_3 : xbsIndex_r4/ROM  depth=128  initVector=cos(2*pi*(256:383)/512)  distributed_mem=Block RAM  rst=off  init_reg=0  en=off  latency=1  gui_display_data_type=Fixed-point  arith_type="Signed  (2's comp)"  n_bits=16  bin_pt=14  preci_type=Single  exp_width=8  frac_width=24  optimize=Area  use_rpm=on  dbl_ovrd=off  block_type=sprom
  ImO0 : Outport
  ReO0 : Outport  Port=2
  dbldout : Outport  Port=3
  syncout : Outport  Port=4
  InO1 : Outport  Port=5
  ReO1 : Outport  Port=6
  ImO2 : Outport  Port=7
  ReO2 : Outport  Port=8
  ImO3 : Outport  Port=9
  ReO3 : Outport  Port=10
  wires:
  Delay1/1 -> Butterfly2/2(ReInOne), Butterfly/2(ReInOne)
  FFT_DIT256_1/1(OutIm0) -> Delay4/1
  In1/1 -> FFT_DIT256_1/1(Im0)
  Butterfly1/2(ReOut) -> ReO1/1
  FFT_DIT256_/3(OutRe0) -> Delay1/1
  FFT_DIT256_/2(dvld) -> Delay8/1, cnt7bit_/2
  Butterfly2/1(Imut) -> ImO2/1
  Delay3/1 -> Butterfly3/2(ReInOne), Butterfly1/2(ReInOne)
  In3/1 -> FFT_DIT256_1/3(Im1)
  retwitddle_1/1 -> Butterfly1/6(TwRe)
  dvldin/1 -> FFT_DIT256_1/6(dvldin), FFT_DIT256_/6(dvldin)
  FFT_DIT256_1/3(OutRe0) -> Delay5/1
  Re3/1 -> FFT_DIT256_1/4(Re1)
  Delay5/1 -> Butterfly2/4(ReInTw), Butterfly/4(ReInTw)
  cnt7bit_/1 -> retwitddle_2/1, imtwiddle_2/1, retwitddle_3/1, imtwiddle_3/1, retwitddle_1/1, imtwiddle_1/1, retwitddle_/1, imtwiddle_/1
  Delay6/1 -> Butterfly3/3(ImInTw), Butterfly1/3(ImInTw)
  imtwiddle_2/1 -> Butterfly3/5(TwIm)
  Delay4/1 -> Butterfly2/3(ImInTw), Butterfly/3(ImInTw)
  retwitddle_2/1 -> Butterfly3/6(TwRe)
  Re2/1 -> FFT_DIT256_/4(Re1)
  Re0/1 -> FFT_DIT256_/2(Re0)
  Butterfly/3(dvldout) -> dbldout/1
  Delay/1 -> Butterfly2/1(ImInOne), Butterfly/1(ImInOne)
  Butterfly3/1(Imut) -> ImO3/1
  retwitddle_3/1 -> Butterfly2/6(TwRe)
  imtwiddle_/1 -> Butterfly/5(TwIm)
  imtwiddle_3/1 -> Butterfly2/5(TwIm)
  FFT_DIT256_/1(OutIm0) -> Delay/1
  Butterfly3/2(ReOut) -> ReO3/1
  Butterfly/1(Imut) -> ImO0/1
  Butterfly/2(ReOut) -> ReO0/1
  FFT_DIT256_1/6(OutRe1) -> Delay7/1
  Delay9/1 -> Butterfly/8(syncin), Butterfly1/8(syncin), Butterfly3/8(syncin), Butterfly2/8(syncin)
  FFT_DIT256_1/5(OutIm1) -> Delay6/1
  Butterfly1/1(Imut) -> InO1/1
  imtwiddle_1/1 -> Butterfly1/5(TwIm)
  Re1/1 -> FFT_DIT256_1/2(Re0)
  Butterfly/4(syncout) -> syncout/1
  FFT_DIT256_/6(OutRe1) -> Delay3/1
  In0/1 -> FFT_DIT256_/1(Im0)
  Delay7/1 -> Butterfly3/4(ReInTw), Butterfly1/4(ReInTw)
  Butterfly2/2(ReOut) -> ReO2/1
  FFT_DIT256_/4(syncout) -> Delay9/1, cnt7bit_/1
  Delay8/1 -> Butterfly/7(dvld), Butterfly1/7(dvld), Butterfly3/7(dvld), Butterfly2/7(dvld)
  FFT_DIT256_/5(OutIm1) -> Delay2/1
  retwitddle_/1 -> Butterfly/6(TwRe)
  In2/1 -> FFT_DIT256_/3(Im1)
  syncin/1 -> FFT_DIT256_1/5(syncin), FFT_DIT256_/5(syncin)
  Delay2/1 -> Butterfly3/1(ImInOne), Butterfly1/1(ImInOne)
  rstn/1 -> FFT_DIT256_1/7(rstn), FFT_DIT256_/7(rstn)
  shift/1 -> FFT_DIT256_1/8(shift), FFT_DIT256_/8(shift)

== system tesv/FFT1024_8_1/Twiddle ==
  Addr : Inport
  imtwiddle_ : xbsIndex_r4/ROM  depth=TFL/NS  initVector="-sin(2*pi*( (WS*TFL/NS) :(  (WS*TFL/NS)+(TFL/NS) -1  ))/TFL)"  distributed_mem=Block RAM  rst=off  init_reg=0  en=off  latency=1  gui_display_data_type=Fixed-point  arith_type="Signed  (2's comp)"  n_bits=16  bin_pt=15  preci_type=Single  exp_width=8  frac_width=24  optimize=Area  use_rpm=on  dbl_ovrd=off  block_type=sprom
  retwitddle_ : xbsIndex_r4/ROM  depth=TFL/NS  initVector="cos(2*pi*( (WS*TFL/NS) :(  (WS*TFL/NS)+(TFL/NS) -1  ))/TFL)"  distributed_mem=Block RAM  rst=off  init_reg=0  en=off  latency=1  gui_display_data_type=Fixed-point  arith_type="Signed  (2's comp)"  n_bits=16  bin_pt=14  preci_type=Single  exp_width=8  frac_width=24  optimize=Area  use_rpm=on  dbl_ovrd=off  block_type=sprom
  IM : Outport
  Re : Outport  Port=2
  wires:
  imtwiddle_/1 -> IM/1
  retwitddle_/1 -> Re/1
  Addr/1 -> retwitddle_/1, imtwiddle_/1

== system tesv/FFT1024_8_1/Twiddle1 ==
  Addr : Inport
  imtwiddle_ : xbsIndex_r4/ROM  depth=TFL/NS  initVector="-sin(2*pi*( (WS*TFL/NS) :(  (WS*TFL/NS)+(TFL/NS) -1  ))/TFL)"  distributed_mem=Block RAM  rst=off  init_reg=0  en=off  latency=1  gui_display_data_type=Fixed-point  arith_type="Signed  (2's comp)"  n_bits=16  bin_pt=15  preci_type=Single  exp_width=8  frac_width=24  optimize=Area  use_rpm=on  dbl_ovrd=off  block_type=sprom
  retwitddle_ : xbsIndex_r4/ROM  depth=TFL/NS  initVector="cos(2*pi*( (WS*TFL/NS) :(  (WS*TFL/NS)+(TFL/NS) -1  ))/TFL)"  distributed_mem=Block RAM  rst=off  init_reg=0  en=off  latency=1  gui_display_data_type=Fixed-point  arith_type="Signed  (2's comp)"  n_bits=16  bin_pt=14  preci_type=Single  exp_width=8  frac_width=24  optimize=Area  use_rpm=on  dbl_ovrd=off  block_type=sprom
  IM : Outport
  Re : Outport  Port=2
  wires:
  imtwiddle_/1 -> IM/1
  retwitddle_/1 -> Re/1
  Addr/1 -> retwitddle_/1, imtwiddle_/1

== system tesv/FFT1024_8_1/Twiddle2 ==
  Addr : Inport
  imtwiddle_ : xbsIndex_r4/ROM  depth=TFL/NS  initVector="-sin(2*pi*( (WS*TFL/NS) :(  (WS*TFL/NS)+(TFL/NS) -1  ))/TFL)"  distributed_mem=Block RAM  rst=off  init_reg=0  en=off  latency=1  gui_display_data_type=Fixed-point  arith_type="Signed  (2's comp)"  n_bits=16  bin_pt=15  preci_type=Single  exp_width=8  frac_width=24  optimize=Area  use_rpm=on  dbl_ovrd=off  block_type=sprom
  retwitddle_ : xbsIndex_r4/ROM  depth=TFL/NS  initVector="cos(2*pi*( (WS*TFL/NS) :(  (WS*TFL/NS)+(TFL/NS) -1  ))/TFL)"  distributed_mem=Block RAM  rst=off  init_reg=0  en=off  latency=1  gui_display_data_type=Fixed-point  arith_type="Signed  (2's comp)"  n_bits=16  bin_pt=14  preci_type=Single  exp_width=8  frac_width=24  optimize=Area  use_rpm=on  dbl_ovrd=off  block_type=sprom
  IM : Outport
  Re : Outport  Port=2
  wires:
  imtwiddle_/1 -> IM/1
  retwitddle_/1 -> Re/1
  Addr/1 -> retwitddle_/1, imtwiddle_/1

== system tesv/FFT1024_8_1/Twiddle3 ==
  Addr : Inport
  imtwiddle_ : xbsIndex_r4/ROM  depth=TFL/NS  initVector="-sin(2*pi*( (WS*TFL/NS) :(  (WS*TFL/NS)+(TFL/NS) -1  ))/TFL)"  distributed_mem=Block RAM  rst=off  init_reg=0  en=off  latency=1  gui_display_data_type=Fixed-point  arith_type="Signed  (2's comp)"  n_bits=16  bin_pt=15  preci_type=Single  exp_width=8  frac_width=24  optimize=Area  use_rpm=on  dbl_ovrd=off  block_type=sprom
  retwitddle_ : xbsIndex_r4/ROM  depth=TFL/NS  initVector="cos(2*pi*( (WS*TFL/NS) :(  (WS*TFL/NS)+(TFL/NS) -1  ))/TFL)"  distributed_mem=Block RAM  rst=off  init_reg=0  en=off  latency=1  gui_display_data_type=Fixed-point  arith_type="Signed  (2's comp)"  n_bits=16  bin_pt=14  preci_type=Single  exp_width=8  frac_width=24  optimize=Area  use_rpm=on  dbl_ovrd=off  block_type=sprom
  IM : Outport
  Re : Outport  Port=2
  wires:
  imtwiddle_/1 -> IM/1
  retwitddle_/1 -> Re/1
  Addr/1 -> retwitddle_/1, imtwiddle_/1

== system tesv/FFT1024_8_1/Twiddle4 ==
  Addr : Inport
  imtwiddle_ : xbsIndex_r4/ROM  depth=TFL/NS  initVector="-sin(2*pi*( (WS*TFL/NS) :(  (WS*TFL/NS)+(TFL/NS) -1  ))/TFL)"  distributed_mem=Block RAM  rst=off  init_reg=0  en=off  latency=1  gui_display_data_type=Fixed-point  arith_type="Signed  (2's comp)"  n_bits=16  bin_pt=15  preci_type=Single  exp_width=8  frac_width=24  optimize=Area  use_rpm=on  dbl_ovrd=off  block_type=sprom
  retwitddle_ : xbsIndex_r4/ROM  depth=TFL/NS  initVector="cos(2*pi*( (WS*TFL/NS) :(  (WS*TFL/NS)+(TFL/NS) -1  ))/TFL)"  distributed_mem=Block RAM  rst=off  init_reg=0  en=off  latency=1  gui_display_data_type=Fixed-point  arith_type="Signed  (2's comp)"  n_bits=16  bin_pt=14  preci_type=Single  exp_width=8  frac_width=24  optimize=Area  use_rpm=on  dbl_ovrd=off  block_type=sprom
  IM : Outport
  Re : Outport  Port=2
  wires:
  imtwiddle_/1 -> IM/1
  retwitddle_/1 -> Re/1
  Addr/1 -> retwitddle_/1, imtwiddle_/1

== system tesv/FFT1024_8_1/Twiddle5 ==
  Addr : Inport
  imtwiddle_ : xbsIndex_r4/ROM  depth=TFL/NS  initVector="-sin(2*pi*( (WS*TFL/NS) :(  (WS*TFL/NS)+(TFL/NS) -1  ))/TFL)"  distributed_mem=Block RAM  rst=off  init_reg=0  en=off  latency=1  gui_display_data_type=Fixed-point  arith_type="Signed  (2's comp)"  n_bits=16  bin_pt=15  preci_type=Single  exp_width=8  frac_width=24  optimize=Area  use_rpm=on  dbl_ovrd=off  block_type=sprom
  retwitddle_ : xbsIndex_r4/ROM  depth=TFL/NS  initVector="cos(2*pi*( (WS*TFL/NS) :(  (WS*TFL/NS)+(TFL/NS) -1  ))/TFL)"  distributed_mem=Block RAM  rst=off  init_reg=0  en=off  latency=1  gui_display_data_type=Fixed-point  arith_type="Signed  (2's comp)"  n_bits=16  bin_pt=14  preci_type=Single  exp_width=8  frac_width=24  optimize=Area  use_rpm=on  dbl_ovrd=off  block_type=sprom
  IM : Outport
  Re : Outport  Port=2
  wires:
  imtwiddle_/1 -> IM/1
  retwitddle_/1 -> Re/1
  Addr/1 -> retwitddle_/1, imtwiddle_/1

== system tesv/FFT1024_8_1/Twiddle6 ==
  Addr : Inport
  imtwiddle_ : xbsIndex_r4/ROM  depth=TFL/NS  initVector="-sin(2*pi*( (WS*TFL/NS) :(  (WS*TFL/NS)+(TFL/NS) -1  ))/TFL)"  distributed_mem=Block RAM  rst=off  init_reg=0  en=off  latency=1  gui_display_data_type=Fixed-point  arith_type="Signed  (2's comp)"  n_bits=16  bin_pt=15  preci_type=Single  exp_width=8  frac_width=24  optimize=Area  use_rpm=on  dbl_ovrd=off  block_type=sprom
  retwitddle_ : xbsIndex_r4/ROM  depth=TFL/NS  initVector="cos(2*pi*( (WS*TFL/NS) :(  (WS*TFL/NS)+(TFL/NS) -1  ))/TFL)"  distributed_mem=Block RAM  rst=off  init_reg=0  en=off  latency=1  gui_display_data_type=Fixed-point  arith_type="Signed  (2's comp)"  n_bits=16  bin_pt=14  preci_type=Single  exp_width=8  frac_width=24  optimize=Area  use_rpm=on  dbl_ovrd=off  block_type=sprom
  IM : Outport
  Re : Outport  Port=2
  wires:
  imtwiddle_/1 -> IM/1
  retwitddle_/1 -> Re/1
  Addr/1 -> retwitddle_/1, imtwiddle_/1

== system tesv/FFT1024_8_1/Twiddle7 ==
  Addr : Inport
  imtwiddle_ : xbsIndex_r4/ROM  depth=TFL/NS  initVector="-sin(2*pi*( (WS*TFL/NS) :(  (WS*TFL/NS)+(TFL/NS) -1  ))/TFL)"  distributed_mem=Block RAM  rst=off  init_reg=0  en=off  latency=1  gui_display_data_type=Fixed-point  arith_type="Signed  (2's comp)"  n_bits=16  bin_pt=15  preci_type=Single  exp_width=8  frac_width=24  optimize=Area  use_rpm=on  dbl_ovrd=off  block_type=sprom
  retwitddle_ : xbsIndex_r4/ROM  depth=TFL/NS  initVector="cos(2*pi*( (WS*TFL/NS) :(  (WS*TFL/NS)+(TFL/NS) -1  ))/TFL)"  distributed_mem=Block RAM  rst=off  init_reg=0  en=off  latency=1  gui_display_data_type=Fixed-point  arith_type="Signed  (2's comp)"  n_bits=16  bin_pt=14  preci_type=Single  exp_width=8  frac_width=24  optimize=Area  use_rpm=on  dbl_ovrd=off  block_type=sprom
  IM : Outport
  Re : Outport  Port=2
  wires:
  imtwiddle_/1 -> IM/1
  retwitddle_/1 -> Re/1
  Addr/1 -> retwitddle_/1, imtwiddle_/1

== system tesv/PFBT2_/CoefAddr_ ==
  sync : Inport
  Iin : Inport  Port=2
  Qin : Inport  Port=3
  Counter : xbsIndex_r4/Counter  cnt_type=Free Running  cnt_to=Inf  operation=Up  start_count=0  cnt_by_val=1  arith_type=Unsigned  n_bits=log2(FL/NS)  bin_pt=0  load_pin=off  rst=on  en=off  explicit_period=on  period=1  use_behavioral_HDL=off  implementation=Fabric  dbl_ovrd=off  block_type=counter
  Delay : xbsIndex_r4/Delay  rst=off  infoeditControl=Selection of Reset will increase slice count due to use of real FFs and instead of SRLs  en=off  latency=1  reg_retiming=off  dbl_ovrd=off  block_type=delay
  Delay1 : xbsIndex_r4/Delay  rst=off  infoeditControl=Selection of Reset will increase slice count due to use of real FFs and instead of SRLs  en=off  latency=1  reg_retiming=off  dbl_ovrd=off  block_type=delay
  Delay2 : xbsIndex_r4/Delay  rst=off  infoeditControl=Selection of Reset will increase slice count due to use of real FFs and instead of SRLs  en=off  latency=1  reg_retiming=off  dbl_ovrd=off  block_type=delay
  Addr : Outport
  Iout : Outport  Port=2
  Qout : Outport  Port=3
  syncout : Outport  Port=4
  wires:
  Counter/1 -> Addr/1
  sync/1 -> Delay2/1, Counter/1
  Iin/1 -> Delay/1
  Qin/1 -> Delay1/1
  Delay/1 -> Iout/1
  Delay1/1 -> Qout/1
  Delay2/1 -> syncout/1

== system tesv/PFBT2_/Delay_ ==
  Iin : Inport
  Qin : Inport  Port=2
  addrin : Inport  Port=3
  sync : Inport  Port=4
  Delay{,1..3} (4 alike) : xbsIndex_r4/Delay  rst=off  infoeditControl=Selection of Reset will increase slice count due to use of real FFs and instead of SRLs  en=off  latency=FL/NS  reg_retiming=off  dbl_ovrd=off  block_type=delay
  Iout : Outport
  Qout : Outport  Port=2
  addrout : Outport  Port=3
  syncout : Outport  Port=4
  wires:
  Iin/1 -> Delay/1
  Delay/1 -> Iout/1
  Delay1/1 -> Qout/1
  Qin/1 -> Delay1/1
  Delay2/1 -> addrout/1
  addrin/1 -> Delay2/1
  Delay3/1 -> syncout/1
  sync/1 -> Delay3/1

== system tesv/PFBT2_/Delay_1 ==
  Iin : Inport
  Qin : Inport  Port=2
  addrin : Inport  Port=3
  sync : Inport  Port=4
  Delay{,1..3} (4 alike) : xbsIndex_r4/Delay  rst=off  infoeditControl=Selection of Reset will increase slice count due to use of real FFs and instead of SRLs  en=off  latency=FL/NS  reg_retiming=off  dbl_ovrd=off  block_type=delay
  Iout : Outport
  Qout : Outport  Port=2
  addrout : Outport  Port=3
  syncout : Outport  Port=4
  wires:
  Iin/1 -> Delay/1
  Delay/1 -> Iout/1
  Delay1/1 -> Qout/1
  Qin/1 -> Delay1/1
  Delay2/1 -> addrout/1
  addrin/1 -> Delay2/1
  Delay3/1 -> syncout/1
  sync/1 -> Delay3/1

== system tesv/PFBT2_/TapIQ_1 ==
  Iin : Inport
  Qin : Inport  Port=2
  coefaddr : Inport  Port=3
  sync : Inport  Port=4
  Delay : xbsIndex_r4/Delay  rst=off  infoeditControl=Selection of Reset will increase slice count due to use of real FFs and instead of SRLs  en=off  latency=FL/NS - 3  reg_retiming=off  dbl_ovrd=off  block_type=delay
  Delay1 : xbsIndex_r4/Delay  rst=off  infoeditControl=Selection of Reset will increase slice count due to use of real FFs and instead of SRLs  en=off  latency=FL/NS -3  reg_retiming=off  dbl_ovrd=off  block_type=delay
  Delay2 : xbsIndex_r4/Delay  rst=off  infoeditControl=Selection of Reset will increase slice count due to use of real FFs and instead of SRLs  en=off  latency=FL/NS -4  reg_retiming=off  dbl_ovrd=off  block_type=delay
  Delay3 : xbsIndex_r4/Delay  rst=off  infoeditControl=Selection of Reset will increase slice count due to use of real FFs and instead of SRLs  en=off  latency=4  reg_retiming=off  dbl_ovrd=off  block_type=delay
  Delay4 : xbsIndex_r4/Delay  rst=off  infoeditControl=Selection of Reset will increase slice count due to use of real FFs and instead of SRLs  en=off  latency=FL/NS  reg_retiming=off  dbl_ovrd=off  block_type=delay
  Mult : xbsIndex_r4/Mult  precision=User Defined  arith_type="Signed  (2's comp)"  n_bits=18  bin_pt=16  quantization=Truncate  overflow=Wrap  en=off  latency=3  use_behavioral_HDL=off  opt=Speed  use_embedded=on  optimum_pipeline=off  pipeline=on  dbl_ovrd=off  use_rpm=on  placement_style=Triangular  block_type=mult
  Mult1 : xbsIndex_r4/Mult  precision=User Defined  arith_type="Signed  (2's comp)"  n_bits=18  bin_pt=16  quantization=Truncate  overflow=Wrap  en=off  latency=3  use_behavioral_HDL=off  opt=Speed  use_embedded=on  optimum_pipeline=off  pipeline=on  dbl_ovrd=off  use_rpm=on  placement_style=Triangular  block_type=mult
  ROM : xbsIndex_r4/ROM  depth=FL/NS  initVector="0.5 - 0.5*cos((2*pi * WT/NT) +  (2*pi/NT)*(WS:NS:(FL-1))/FL)"  distributed_mem=Block RAM  rst=off  init_reg=0  en=off  latency=1  gui_display_data_type=Fixed-point  arith_type="Signed  (2's comp)"  n_bits=18  bin_pt=16  preci_type=Single  exp_width=8  frac_width=24  optimize=Area  use_rpm=on  dbl_ovrd=off  block_type=sprom
  Iout : Outport
  Qout : Outport  Port=2
  coefaddrout : Outport  Port=3
  syncout : Outport  Port=4
  wires:
  Qin/1 -> Delay1/1
  ROM/1 -> Mult1/2, Mult/2
  Mult/1 -> Iout/1
  coefaddr/1 -> Delay2/1
  Mult1/1 -> Qout/1
  Iin/1 -> Delay/1
  Delay/1 -> Mult/1
  Delay1/1 -> Mult1/1
  Delay2/1 -> Delay3/1, ROM/1
  Delay3/1 -> coefaddrout/1
  sync/1 -> Delay4/1
  Delay4/1 -> syncout/1

== system tesv/PFBT2_/TapIQ_2 ==
  Iin : Inport
  Qin : Inport  Port=2
  coefaddr : Inport  Port=3
  sync : Inport  Port=4
  Delay : xbsIndex_r4/Delay  rst=off  infoeditControl=Selection of Reset will increase slice count due to use of real FFs and instead of SRLs  en=off  latency=FL/NS - 3  reg_retiming=off  dbl_ovrd=off  block_type=delay
  Delay1 : xbsIndex_r4/Delay  rst=off  infoeditControl=Selection of Reset will increase slice count due to use of real FFs and instead of SRLs  en=off  latency=FL/NS -3  reg_retiming=off  dbl_ovrd=off  block_type=delay
  Delay2 : xbsIndex_r4/Delay  rst=off  infoeditControl=Selection of Reset will increase slice count due to use of real FFs and instead of SRLs  en=off  latency=FL/NS -4  reg_retiming=off  dbl_ovrd=off  block_type=delay
  Delay3 : xbsIndex_r4/Delay  rst=off  infoeditControl=Selection of Reset will increase slice count due to use of real FFs and instead of SRLs  en=off  latency=4  reg_retiming=off  dbl_ovrd=off  block_type=delay
  Delay4 : xbsIndex_r4/Delay  rst=off  infoeditControl=Selection of Reset will increase slice count due to use of real FFs and instead of SRLs  en=off  latency=FL/NS  reg_retiming=off  dbl_ovrd=off  block_type=delay
  Mult : xbsIndex_r4/Mult  precision=User Defined  arith_type="Signed  (2's comp)"  n_bits=18  bin_pt=16  quantization=Truncate  overflow=Wrap  en=off  latency=3  use_behavioral_HDL=off  opt=Speed  use_embedded=on  optimum_pipeline=off  pipeline=on  dbl_ovrd=off  use_rpm=on  placement_style=Triangular  block_type=mult
  Mult1 : xbsIndex_r4/Mult  precision=User Defined  arith_type="Signed  (2's comp)"  n_bits=18  bin_pt=16  quantization=Truncate  overflow=Wrap  en=off  latency=3  use_behavioral_HDL=off  opt=Speed  use_embedded=on  optimum_pipeline=off  pipeline=on  dbl_ovrd=off  use_rpm=on  placement_style=Triangular  block_type=mult
  ROM : xbsIndex_r4/ROM  depth=FL/NS  initVector="0.5 - 0.5*cos((2*pi * WT/NT) +  (2*pi/NT)*(WS:NS:(FL-1))/FL)"  distributed_mem=Block RAM  rst=off  init_reg=0  en=off  latency=1  gui_display_data_type=Fixed-point  arith_type="Signed  (2's comp)"  n_bits=18  bin_pt=16  preci_type=Single  exp_width=8  frac_width=24  optimize=Area  use_rpm=on  dbl_ovrd=off  block_type=sprom
  Iout : Outport
  Qout : Outport  Port=2
  coefaddrout : Outport  Port=3
  syncout : Outport  Port=4
  wires:
  Qin/1 -> Delay1/1
  ROM/1 -> Mult1/2, Mult/2
  Mult/1 -> Iout/1
  coefaddr/1 -> Delay2/1
  Mult1/1 -> Qout/1
  Iin/1 -> Delay/1
  Delay/1 -> Mult/1
  Delay1/1 -> Mult1/1
  Delay2/1 -> Delay3/1, ROM/1
  Delay3/1 -> coefaddrout/1
  sync/1 -> Delay4/1
  Delay4/1 -> syncout/1

== system tesv/PFBT2_1/CoefAddr_ ==
  sync : Inport
  Iin : Inport  Port=2
  Qin : Inport  Port=3
  Counter : xbsIndex_r4/Counter  cnt_type=Free Running  cnt_to=Inf  operation=Up  start_count=0  cnt_by_val=1  arith_type=Unsigned  n_bits=log2(FL/NS)  bin_pt=0  load_pin=off  rst=on  en=off  explicit_period=on  period=1  use_behavioral_HDL=off  implementation=Fabric  dbl_ovrd=off  block_type=counter
  Delay : xbsIndex_r4/Delay  rst=off  infoeditControl=Selection of Reset will increase slice count due to use of real FFs and instead of SRLs  en=off  latency=1  reg_retiming=off  dbl_ovrd=off  block_type=delay
  Delay1 : xbsIndex_r4/Delay  rst=off  infoeditControl=Selection of Reset will increase slice count due to use of real FFs and instead of SRLs  en=off  latency=1  reg_retiming=off  dbl_ovrd=off  block_type=delay
  Delay2 : xbsIndex_r4/Delay  rst=off  infoeditControl=Selection of Reset will increase slice count due to use of real FFs and instead of SRLs  en=off  latency=1  reg_retiming=off  dbl_ovrd=off  block_type=delay
  Addr : Outport
  Iout : Outport  Port=2
  Qout : Outport  Port=3
  syncout : Outport  Port=4
  wires:
  Counter/1 -> Addr/1
  sync/1 -> Delay2/1, Counter/1
  Iin/1 -> Delay/1
  Qin/1 -> Delay1/1
  Delay/1 -> Iout/1
  Delay1/1 -> Qout/1
  Delay2/1 -> syncout/1

== system tesv/PFBT2_1/Delay_ ==
  Iin : Inport
  Qin : Inport  Port=2
  addrin : Inport  Port=3
  sync : Inport  Port=4
  Delay{,1..3} (4 alike) : xbsIndex_r4/Delay  rst=off  infoeditControl=Selection of Reset will increase slice count due to use of real FFs and instead of SRLs  en=off  latency=FL/NS  reg_retiming=off  dbl_ovrd=off  block_type=delay
  Iout : Outport
  Qout : Outport  Port=2
  addrout : Outport  Port=3
  syncout : Outport  Port=4
  wires:
  Iin/1 -> Delay/1
  Delay/1 -> Iout/1
  Delay1/1 -> Qout/1
  Qin/1 -> Delay1/1
  Delay2/1 -> addrout/1
  addrin/1 -> Delay2/1
  Delay3/1 -> syncout/1
  sync/1 -> Delay3/1
